simulink model "OML58_Cores2"  (R2021b)
settings: Solver=ode1  StartTime=0.0  StopTime=10  FixedStep=Ts  RelTol=1e-3
PostLoadFcn:
  | Ts = 50e-6;
InitFcn:
  | Ts = 50e-6;
undefined symbols (not defined in the file): I, Left, Right, type, V, X
libraries: spsSeriesRLCBranchLib x30, artemis x20, spsThreePhaseSeriesRLCBranchLib x19, spsThreePhaseSeriesRLCLoadLib x15, spsThreePhaseBreakerLib x15, spsGroundLib x12, rtlab x9, LafaeLib x8, spsThreePhaseVIMeasurementLib x7, spsThreePhaseTransformerTwoWindingsLib x5, spsPower3phInstantaneousLib x5, spsStairGeneratorLib x2
(part 3 of 3)

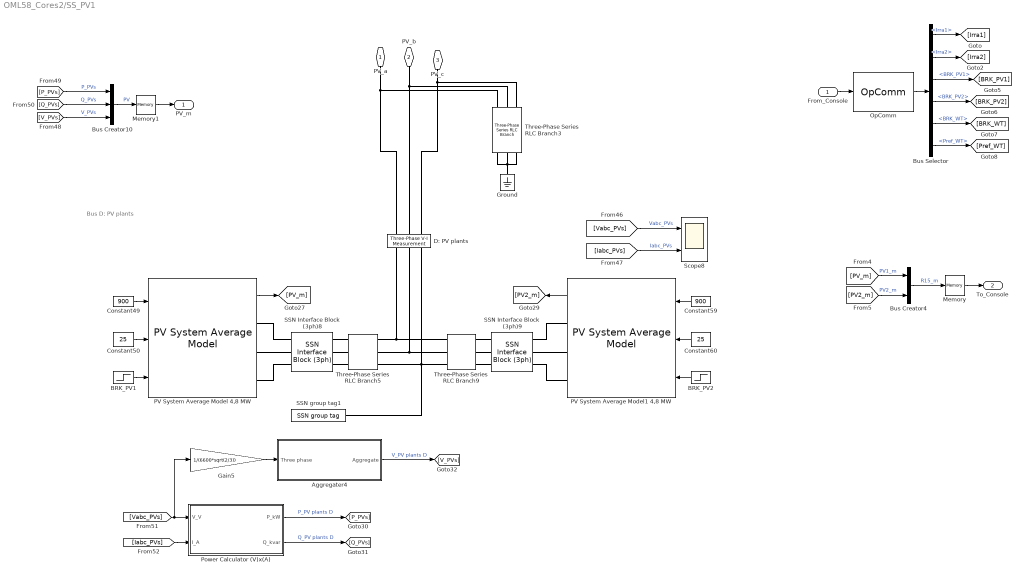
== system OML58_Cores2/SS_PV1 ==
  note: Bus D: PV plants
  From_Console : Inport
  Aggregater4 : Subsystem
      mask Display: image('$imagefile'); % Use "Edit Image" on toolstrip to change.
  BRK_PV1 : Step  Time=40  SampleTime=0
  BRK_PV2 : Step  Time=45  SampleTime=0
  Bus Creator10 : BusCreator  Inputs=3
  Bus Creator4 : BusCreator  Inputs=2
  Bus Selector : BusSelector  OutputSignals=Irra1,Irra2,BRK_PV1,BRK_PV2,BRK_WT,Pref_WT
  Constant49 : Constant  Value=900
  Constant50 : Constant  Value=25
  Constant59 : Constant  Value=900
  Constant60 : Constant  Value=25
  D: PV plants : spsThreePhaseVIMeasurementLib/Three-Phase V-I Measurement  VoltageMeasurement=phase-to-ground  SetLabelV=on  LabelV=Vabc_PVs  Vpu=off  VpuLL=off  CurrentMeasurement=yes  SetLabelI=on  LabelI=Iabc_PVs  Ipu=off  Pbase=100e6  Vbase=500e3  OutputType=Magnitude  PhasorSimulation=off  PSBequivalent=0
  Gain5 : Gain  Gain=1/(6600*sqrt(2/3))
  Ground : spsGroundLib/Ground  LConnTagsString=a
  Memory : Memory
  Memory1 : Memory
  OpComm : rtlab/OpComm  nbport=1  groupe_acq=1  subsys_rate=0  st=0  Synchronization=on  Interpolation=on  Threshold=1.0  Missed_Data=off  Sim_Time=off  Samples=off  dynSigOut=off  from_console=1  warning_done=off  writeOpCommFile=off  Offset=off
      settings: SourceProductName=RT-LAB
  PV System Average Model 4,8 MW : LafaeLib/PV System/PV System Average Model  Pnom=4.8e6  PF=1  fnom=50  Vdc_ref=1500  fsw=3*42*50  ripple_c=0.05  R1=0.001  Vdc_mpp=820.5  ripple_i_Boost=0.05  ripple_v_Boost=0.05  Vca_trafo_high=6.6e3  Vrms_high=6.6e3  Vrms_low=690  X_pu_trafo=0.1  tau_i=1e-3  Ts=Ts  Ts_Control=2*Ts
      link override PV Array: Npar=Np
      settings: SourceProductName=LAFAE Library
  PV System Average Model1 4,8 MW : LafaeLib/PV System/PV System Average Model  Pnom=4.8e6  PF=1  fnom=50  Vdc_ref=1500  fsw=3*42*50  ripple_c=0.05  R1=0.001  Vdc_mpp=820.5  ripple_i_Boost=0.05  ripple_v_Boost=0.05  Vca_trafo_high=6.6e3  Vrms_high=6.6e3  Vrms_low=690  X_pu_trafo=0.1  tau_i=1e-3  Ts=Ts  Ts_Control=2*Ts
      link override PV Array: Npar=Np
      settings: SourceProductName=LAFAE Library
  Power Calculator (V)x(A) : Subsystem
      mask DialogControl DescTextVar Prompt: Compute the three-phase instantaneous active and reactive powers associated with a periodic set of three-phase voltages and currents.
      mask DialogControl Control2 Prompt: Instantaneous reactive power is accurate only for balanced and harmonic-free three-phase voltages and currents.
      mask DialogControl Control3 Prompt: Current flowing into an RL circuit will produce positive active and reactive power.
      mask DialogControl Control4 Prompt: Input currents and voltages in (A) and (V), respectively.
      mask DialogControl Control5 Prompt: Output P and Q in kW and kvar, respectively.
      mask Display: image('$imagefile'); % Use "Edit Image" on toolstrip to change.
  SSN Interface Block (3ph)8 : artemis/SSN/Nodal Interface Blocks/SSN Interface Block (3ph)  nb_phase=3  nb_port=2  p1_type=I-type(Left)  p2_type=V-type (Right)  p3_type=V-type(Left)  p4_type=V-type(Left)  p5_type=V-type(Left)  p6_type=V-type(Left)  p7_type=V-type(Left)  p8_type=V-type(Left)  p9_type=V-type(Left)  p10_type=V-type(Left)  p11_type=V-type(Left)  p12_type=V-type(Left)  p13_type=V-type(Left)  p14_type=V-type(Left)  p15_type=V-type(Left)  p16_type=V-type(Left)  I_port_shunt_resistance=1e6
  SSN Interface Block (3ph)9 : artemis/SSN/Nodal Interface Blocks/SSN Interface Block (3ph)  nb_phase=3  nb_port=2  p1_type=V-type(Left)  p2_type=V-type (Right)  p3_type=V-type(Left)  p4_type=V-type(Left)  p5_type=V-type(Left)  p6_type=V-type(Left)  p7_type=V-type(Left)  p8_type=V-type(Left)  p9_type=V-type(Left)  p10_type=V-type(Left)  p11_type=V-type(Left)  p12_type=V-type(Left)  p13_type=V-type(Left)  p14_type=V-type(Left)  p15_type=V-type(Left)  p16_type=V-type(Left)  I_port_shunt_resistance=1e6
  SSN group tag1 : artemis/SSN/SSN group tag  ssn_group_tag=PV_Plant
  Scope8 : Scope  NumInputPorts=2
  Three-Phase Series RLC Branch3 : spsThreePhaseSeriesRLCBranchLib/Three-Phase Series RLC Branch  LConnTagsString=A|B|C  RConnTagsString=A|B|C  BranchType=L  Resistance=1  Inductance=2*2.5943  Capacitance=1e-6  Measurements=None
  Three-Phase Series RLC Branch5 : spsThreePhaseSeriesRLCBranchLib/Three-Phase Series RLC Branch  LConnTagsString=A|B|C  RConnTagsString=A|B|C  BranchType=R  Resistance=1e-6  Inductance=1e-3  Capacitance=1e-6  Measurements=None
  Three-Phase Series RLC Branch9 : spsThreePhaseSeriesRLCBranchLib/Three-Phase Series RLC Branch  LConnTagsString=A|B|C  RConnTagsString=A|B|C  BranchType=R  Resistance=1e-6  Inductance=1e-3  Capacitance=1e-6  Measurements=None
  PV_a : PMIOPort  Side=Right
  PV_b : PMIOPort  Port=2  Side=Right
  PV_c : PMIOPort  Port=3  Side=Right
  PV_m : Outport
  To_Console : Outport  Port=2
  wires:
  Memory/1 -> To_Console/1
  From_Console/1 -> OpComm/1
  OpComm/1 -> Bus Selector/1
  Bus Selector/1 -> [Irra1]  "<Irra1>"
  Bus Selector/2 -> [Irra2]  "<Irra2>"
  Bus Selector/3 -> [BRK_PV1]  "<BRK_PV1>"
  Bus Selector/4 -> [BRK_PV2]  "<BRK_PV2>"
  Bus Selector/5 -> [BRK_WT]  "<BRK_WT>"
  Bus Creator4/1 -> Memory/1  "R15_m"
  [PV2_m] -> Bus Creator4/2  "PV2_m"
  [PV_m] -> Bus Creator4/1  "PV1_m"
  Bus Selector/6 -> [Pref_WT]  "<Pref_WT>"
  BRK_PV2/1 -> PV System Average Model1 4,8 MW/3
  [V_PVs] -> Bus Creator10/3  "V_PVs"
  Gain5/1 -> Aggregater4/1(Three phase)
  [Vabc_PVs] -> Power Calculator (V)x(A)/1(V_V), Gain5/1
  Constant49/1 -> PV System Average Model 4,8 MW/1
  [Iabc_PVs] -> Scope8/2  "Iabc_PVs"
  Constant50/1 -> PV System Average Model 4,8 MW/2
  [Iabc_PVs] -> Power Calculator (V)x(A)/2(I_A)
  [Vabc_PVs] -> Scope8/1  "Vabc_PVs"
  Aggregater4/1(Aggregate) -> [V_PVs]  "V_PV plants D"
  Constant59/1 -> PV System Average Model1 4,8 MW/1
  BRK_PV1/1 -> PV System Average Model 4,8 MW/3
  Power Calculator (V)x(A)/2(Q_kvar) -> [Q_PVs]  "Q_PV plants D"
  Memory1/1 -> PV_m/1
  PV System Average Model1 4,8 MW/1 -> [PV2_m]
  Constant60/1 -> PV System Average Model1 4,8 MW/2
  Power Calculator (V)x(A)/1(P_kW) -> [P_PVs]  "P_PV plants D"
  Bus Creator10/1 -> Memory1/1  "PV"
  [P_PVs] -> Bus Creator10/1  "P_PVs"
  PV System Average Model 4,8 MW/1 -> [PV_m]
  [Q_PVs] -> Bus Creator10/2  "Q_PVs"
  connections:
  D: PV plants/RConn1 -- PV_a/RConn1 -- Three-Phase Series RLC Branch3/LConn1
  SSN group tag1/LConn1 -- D: PV plants/LConn3 -- Three-Phase Series RLC Branch5/LConn3 -- Three-Phase Series RLC Branch9/LConn3
  D: PV plants/RConn2 -- PV_b/RConn1 -- Three-Phase Series RLC Branch3/LConn2
  Three-Phase Series RLC Branch3/RConn1 -- Ground/LConn1 -- Three-Phase Series RLC Branch3/RConn2 -- Three-Phase Series RLC Branch3/RConn3
  D: PV plants/RConn3 -- PV_c/RConn1 -- Three-Phase Series RLC Branch3/LConn3
  Three-Phase Series RLC Branch9/LConn2 -- D: PV plants/LConn2 -- Three-Phase Series RLC Branch5/LConn2
  Three-Phase Series RLC Branch9/LConn1 -- D: PV plants/LConn1 -- Three-Phase Series RLC Branch5/LConn1
  Three-Phase Series RLC Branch5/RConn2 -- SSN Interface Block (3ph)8/LConn2
  PV System Average Model 4,8 MW/RConn3 -- SSN Interface Block (3ph)8/RConn3
  PV System Average Model 4,8 MW/RConn2 -- SSN Interface Block (3ph)8/RConn2
  PV System Average Model1 4,8 MW/RConn1 -- SSN Interface Block (3ph)9/LConn1
  SSN Interface Block (3ph)9/RConn1 -- Three-Phase Series RLC Branch9/RConn1
  Three-Phase Series RLC Branch5/RConn1 -- SSN Interface Block (3ph)8/LConn1
  SSN Interface Block (3ph)9/RConn2 -- Three-Phase Series RLC Branch9/RConn2
  SSN Interface Block (3ph)9/RConn3 -- Three-Phase Series RLC Branch9/RConn3
  PV System Average Model 4,8 MW/RConn1 -- SSN Interface Block (3ph)8/RConn1
  PV System Average Model1 4,8 MW/RConn2 -- SSN Interface Block (3ph)9/LConn2
  Three-Phase Series RLC Branch5/RConn3 -- SSN Interface Block (3ph)8/LConn3
  PV System Average Model1 4,8 MW/RConn3 -- SSN Interface Block (3ph)9/LConn3

== system OML58_Cores2/SM_powergrid/Aggregater ==
  Three phase : Inport
  Gain6 : Gain  Gain=2/3
  Sqrt : Sqrt  SaturateOnIntegerOverflow=on
  Square : Math  Operator=square  SaturateOnIntegerOverflow=on
  Sum5 : Sum  Inputs=1  CollapseMode=Specified dimension
  Aggregate : Outport
  wires:
  Gain6/1 -> Sqrt/1
  Sum5/1 -> Gain6/1
  Square/1 -> Sum5/1
  Sqrt/1 -> Aggregate/1
  Three phase/1 -> Square/1

== system OML58_Cores2/SM_powergrid/Aggregater1 ==
  Three phase : Inport
  Gain6 : Gain  Gain=2/3
  Sqrt : Sqrt  SaturateOnIntegerOverflow=on
  Square : Math  Operator=square  SaturateOnIntegerOverflow=on
  Sum5 : Sum  Inputs=1  CollapseMode=Specified dimension
  Aggregate : Outport
  wires:
  Gain6/1 -> Sqrt/1
  Sum5/1 -> Gain6/1
  Square/1 -> Sum5/1
  Sqrt/1 -> Aggregate/1
  Three phase/1 -> Square/1

== system OML58_Cores2/SM_powergrid/Aggregater2 ==
  Three phase : Inport
  Gain6 : Gain  Gain=2/3
  Sqrt : Sqrt  SaturateOnIntegerOverflow=on
  Square : Math  Operator=square  SaturateOnIntegerOverflow=on
  Sum5 : Sum  Inputs=1  CollapseMode=Specified dimension
  Aggregate : Outport
  wires:
  Gain6/1 -> Sqrt/1
  Sum5/1 -> Gain6/1
  Square/1 -> Sum5/1
  Sqrt/1 -> Aggregate/1
  Three phase/1 -> Square/1

== system OML58_Cores2/SM_powergrid/Aggregater3 ==
  Three phase : Inport
  Gain6 : Gain  Gain=2/3
  Sqrt : Sqrt  SaturateOnIntegerOverflow=on
  Square : Math  Operator=square  SaturateOnIntegerOverflow=on
  Sum5 : Sum  Inputs=1  CollapseMode=Specified dimension
  Aggregate : Outport
  wires:
  Gain6/1 -> Sqrt/1
  Sum5/1 -> Gain6/1
  Square/1 -> Sum5/1
  Sqrt/1 -> Aggregate/1
  Three phase/1 -> Square/1

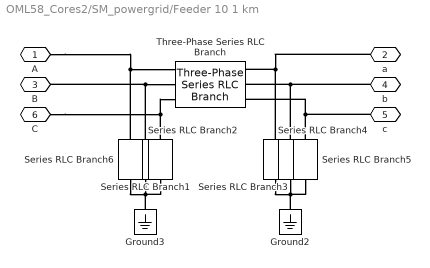
== system OML58_Cores2/SM_powergrid/Feeder 10 1 km ==
  Ground2 : spsGroundLib/Ground  LConnTagsString=a
  Ground3 : spsGroundLib/Ground  LConnTagsString=a
  Series RLC Branch{1..6} (6 alike) : spsSeriesRLCBranchLib/Series RLC Branch  LConnTagsString=__new0  RConnTagsString=__new0  BranchType=C  Resistance=1  Inductance=1e-3  SetiL0=off  InitialCurrent=0  Capacitance=l*0.495e-6/2  Setx0=off  InitialVoltage=0  Measurements=None
  Three-Phase Series RLC Branch : spsThreePhaseSeriesRLCBranchLib/Three-Phase Series RLC Branch  LConnTagsString=A|B|C  RConnTagsString=A|B|C  BranchType=RL  Resistance=l*0.0991  Inductance=l*0.602e-3  Capacitance=1e-6  Measurements=None
  A : PMIOPort  Side=Left
  a : PMIOPort  Port=2  Side=Right
  B : PMIOPort  Port=3  Side=Left
  b : PMIOPort  Port=4  Side=Right
  c : PMIOPort  Port=5  Side=Right
  C : PMIOPort  Port=6  Side=Left
  connections:
  Ground2/LConn1 -- Series RLC Branch5/RConn1 -- Series RLC Branch4/RConn1 -- Series RLC Branch3/RConn1
  Series RLC Branch2/LConn1 -- C/RConn1 -- Three-Phase Series RLC Branch/LConn3
  Ground3/LConn1 -- Series RLC Branch2/RConn1 -- Series RLC Branch1/RConn1 -- Series RLC Branch6/RConn1
  Series RLC Branch3/LConn1 -- a/RConn1 -- Three-Phase Series RLC Branch/RConn1
  Series RLC Branch6/LConn1 -- A/RConn1 -- Three-Phase Series RLC Branch/LConn1
  Series RLC Branch4/LConn1 -- b/RConn1 -- Three-Phase Series RLC Branch/RConn2
  Series RLC Branch5/LConn1 -- c/RConn1 -- Three-Phase Series RLC Branch/RConn3
  Series RLC Branch1/LConn1 -- B/RConn1 -- Three-Phase Series RLC Branch/LConn2

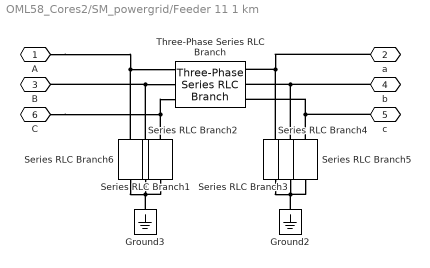
== system OML58_Cores2/SM_powergrid/Feeder 11 1 km ==
  Ground2 : spsGroundLib/Ground  LConnTagsString=a
  Ground3 : spsGroundLib/Ground  LConnTagsString=a
  Series RLC Branch{1..6} (6 alike) : spsSeriesRLCBranchLib/Series RLC Branch  LConnTagsString=__new0  RConnTagsString=__new0  BranchType=C  Resistance=1  Inductance=1e-3  SetiL0=off  InitialCurrent=0  Capacitance=l*0.495e-6/2  Setx0=off  InitialVoltage=0  Measurements=None
  Three-Phase Series RLC Branch : spsThreePhaseSeriesRLCBranchLib/Three-Phase Series RLC Branch  LConnTagsString=A|B|C  RConnTagsString=A|B|C  BranchType=RL  Resistance=l*0.0991  Inductance=l*0.602e-3  Capacitance=1e-6  Measurements=None
  A : PMIOPort  Side=Left
  a : PMIOPort  Port=2  Side=Right
  B : PMIOPort  Port=3  Side=Left
  b : PMIOPort  Port=4  Side=Right
  c : PMIOPort  Port=5  Side=Right
  C : PMIOPort  Port=6  Side=Left
  connections:
  Ground2/LConn1 -- Series RLC Branch5/RConn1 -- Series RLC Branch4/RConn1 -- Series RLC Branch3/RConn1
  Series RLC Branch2/LConn1 -- C/RConn1 -- Three-Phase Series RLC Branch/LConn3
  Ground3/LConn1 -- Series RLC Branch2/RConn1 -- Series RLC Branch1/RConn1 -- Series RLC Branch6/RConn1
  Series RLC Branch3/LConn1 -- a/RConn1 -- Three-Phase Series RLC Branch/RConn1
  Series RLC Branch6/LConn1 -- A/RConn1 -- Three-Phase Series RLC Branch/LConn1
  Series RLC Branch4/LConn1 -- b/RConn1 -- Three-Phase Series RLC Branch/RConn2
  Series RLC Branch5/LConn1 -- c/RConn1 -- Three-Phase Series RLC Branch/RConn3
  Series RLC Branch1/LConn1 -- B/RConn1 -- Three-Phase Series RLC Branch/LConn2

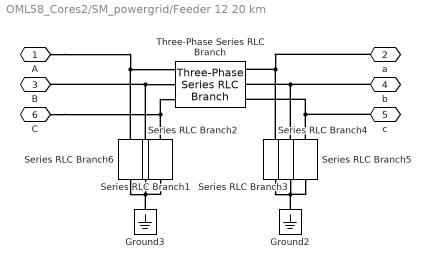
== system OML58_Cores2/SM_powergrid/Feeder 12 20 km ==
  Ground2 : spsGroundLib/Ground  LConnTagsString=a
  Ground3 : spsGroundLib/Ground  LConnTagsString=a
  Series RLC Branch{1..6} (6 alike) : spsSeriesRLCBranchLib/Series RLC Branch  LConnTagsString=__new0  RConnTagsString=__new0  BranchType=C  Resistance=1  Inductance=1e-3  SetiL0=off  InitialCurrent=0  Capacitance=l*0.495e-6/2  Setx0=off  InitialVoltage=0  Measurements=None
  Three-Phase Series RLC Branch : spsThreePhaseSeriesRLCBranchLib/Three-Phase Series RLC Branch  LConnTagsString=A|B|C  RConnTagsString=A|B|C  BranchType=RL  Resistance=l*0.0991  Inductance=l*0.602e-3  Capacitance=1e-6  Measurements=None
  A : PMIOPort  Side=Left
  a : PMIOPort  Port=2  Side=Right
  B : PMIOPort  Port=3  Side=Left
  b : PMIOPort  Port=4  Side=Right
  c : PMIOPort  Port=5  Side=Right
  C : PMIOPort  Port=6  Side=Left
  connections:
  Ground2/LConn1 -- Series RLC Branch5/RConn1 -- Series RLC Branch4/RConn1 -- Series RLC Branch3/RConn1
  Series RLC Branch2/LConn1 -- C/RConn1 -- Three-Phase Series RLC Branch/LConn3
  Ground3/LConn1 -- Series RLC Branch2/RConn1 -- Series RLC Branch1/RConn1 -- Series RLC Branch6/RConn1
  Series RLC Branch3/LConn1 -- a/RConn1 -- Three-Phase Series RLC Branch/RConn1
  Series RLC Branch6/LConn1 -- A/RConn1 -- Three-Phase Series RLC Branch/LConn1
  Series RLC Branch4/LConn1 -- b/RConn1 -- Three-Phase Series RLC Branch/RConn2
  Series RLC Branch5/LConn1 -- c/RConn1 -- Three-Phase Series RLC Branch/RConn3
  Series RLC Branch1/LConn1 -- B/RConn1 -- Three-Phase Series RLC Branch/LConn2

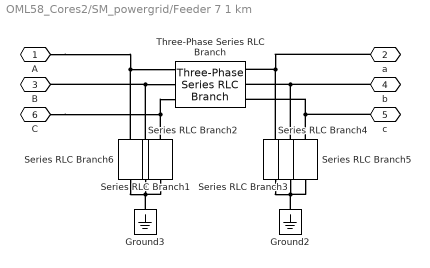
== system OML58_Cores2/SM_powergrid/Feeder 7 1 km ==
  Ground2 : spsGroundLib/Ground  LConnTagsString=a
  Ground3 : spsGroundLib/Ground  LConnTagsString=a
  Series RLC Branch{1..6} (6 alike) : spsSeriesRLCBranchLib/Series RLC Branch  LConnTagsString=__new0  RConnTagsString=__new0  BranchType=C  Resistance=1  Inductance=1e-3  SetiL0=off  InitialCurrent=0  Capacitance=l*0.495e-6/2  Setx0=off  InitialVoltage=0  Measurements=None
  Three-Phase Series RLC Branch : spsThreePhaseSeriesRLCBranchLib/Three-Phase Series RLC Branch  LConnTagsString=A|B|C  RConnTagsString=A|B|C  BranchType=RL  Resistance=l*0.0991  Inductance=l*0.602e-3  Capacitance=1e-6  Measurements=None
  A : PMIOPort  Side=Left
  a : PMIOPort  Port=2  Side=Right
  B : PMIOPort  Port=3  Side=Left
  b : PMIOPort  Port=4  Side=Right
  c : PMIOPort  Port=5  Side=Right
  C : PMIOPort  Port=6  Side=Left
  connections:
  Ground2/LConn1 -- Series RLC Branch5/RConn1 -- Series RLC Branch4/RConn1 -- Series RLC Branch3/RConn1
  Series RLC Branch2/LConn1 -- C/RConn1 -- Three-Phase Series RLC Branch/LConn3
  Ground3/LConn1 -- Series RLC Branch2/RConn1 -- Series RLC Branch1/RConn1 -- Series RLC Branch6/RConn1
  Series RLC Branch3/LConn1 -- a/RConn1 -- Three-Phase Series RLC Branch/RConn1
  Series RLC Branch6/LConn1 -- A/RConn1 -- Three-Phase Series RLC Branch/LConn1
  Series RLC Branch4/LConn1 -- b/RConn1 -- Three-Phase Series RLC Branch/RConn2
  Series RLC Branch5/LConn1 -- c/RConn1 -- Three-Phase Series RLC Branch/RConn3
  Series RLC Branch1/LConn1 -- B/RConn1 -- Three-Phase Series RLC Branch/LConn2

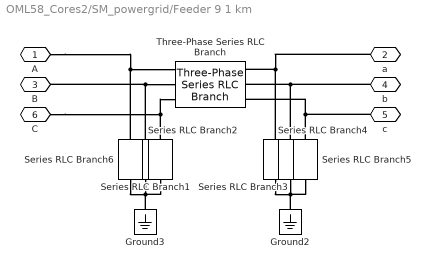
== system OML58_Cores2/SM_powergrid/Feeder 9 1 km ==
  Ground2 : spsGroundLib/Ground  LConnTagsString=a
  Ground3 : spsGroundLib/Ground  LConnTagsString=a
  Series RLC Branch{1..6} (6 alike) : spsSeriesRLCBranchLib/Series RLC Branch  LConnTagsString=__new0  RConnTagsString=__new0  BranchType=C  Resistance=1  Inductance=1e-3  SetiL0=off  InitialCurrent=0  Capacitance=l*0.495e-6/2  Setx0=off  InitialVoltage=0  Measurements=None
  Three-Phase Series RLC Branch : spsThreePhaseSeriesRLCBranchLib/Three-Phase Series RLC Branch  LConnTagsString=A|B|C  RConnTagsString=A|B|C  BranchType=RL  Resistance=l*0.0991  Inductance=l*0.602e-3  Capacitance=1e-6  Measurements=None
  A : PMIOPort  Side=Left
  a : PMIOPort  Port=2  Side=Right
  B : PMIOPort  Port=3  Side=Left
  b : PMIOPort  Port=4  Side=Right
  c : PMIOPort  Port=5  Side=Right
  C : PMIOPort  Port=6  Side=Left
  connections:
  Ground2/LConn1 -- Series RLC Branch5/RConn1 -- Series RLC Branch4/RConn1 -- Series RLC Branch3/RConn1
  Series RLC Branch2/LConn1 -- C/RConn1 -- Three-Phase Series RLC Branch/LConn3
  Ground3/LConn1 -- Series RLC Branch2/RConn1 -- Series RLC Branch1/RConn1 -- Series RLC Branch6/RConn1
  Series RLC Branch3/LConn1 -- a/RConn1 -- Three-Phase Series RLC Branch/RConn1
  Series RLC Branch6/LConn1 -- A/RConn1 -- Three-Phase Series RLC Branch/LConn1
  Series RLC Branch4/LConn1 -- b/RConn1 -- Three-Phase Series RLC Branch/RConn2
  Series RLC Branch5/LConn1 -- c/RConn1 -- Three-Phase Series RLC Branch/RConn3
  Series RLC Branch1/LConn1 -- B/RConn1 -- Three-Phase Series RLC Branch/LConn2

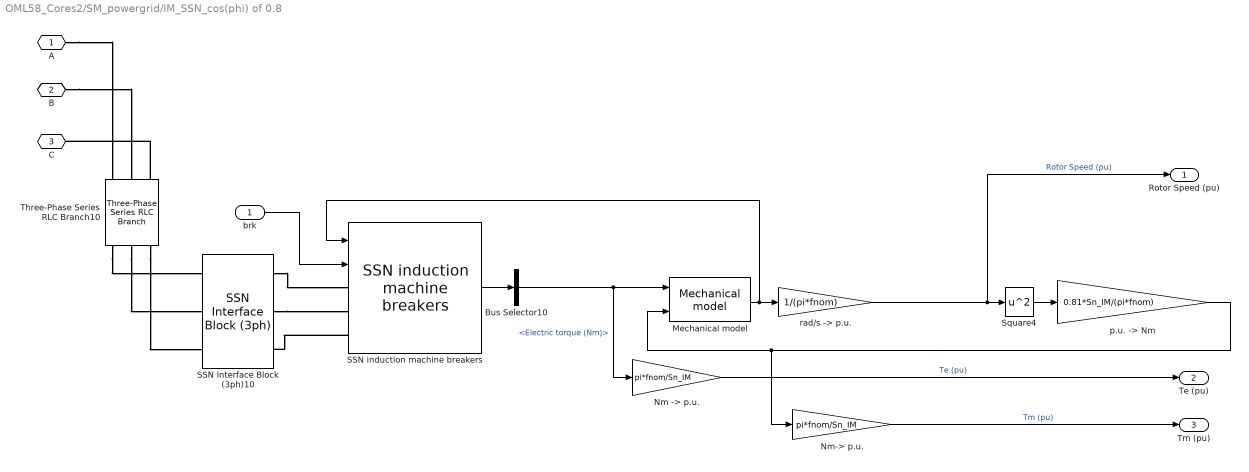
== system OML58_Cores2/SM_powergrid/IM_SSN_cos(phi) of 0.8 ==
  brk : Inport
  Bus Selector10 : BusSelector  OutputSignals=Electric torque (Nm)
  Mechanical model : artemis/SSN/SSN rotating machines/Mechanical model  J=Sn_IM/(fnom*pi)^2  F=6.2988e-004  fo=eps  Ts=Ts
  "Nm -> p.u." : Gain  Gain=pi*fnom/Sn_IM
  Nm-> p.u. : Gain  Gain=pi*fnom/Sn_IM
  SSN Interface Block (3ph)10 : artemis/SSN/Nodal Interface Blocks/SSN Interface Block (3ph)  nb_phase=3  nb_port=2  p1_type=X-type(Right)  p2_type=V-type(Left)  p3_type=V-type(Left)  p4_type=V-type(Left)  p5_type=V-type(Left)  p6_type=V-type(Left)  p7_type=V-type(Left)  p8_type=V-type(Left)  p9_type=V-type(Left)  p10_type=V-type(Left)  p11_type=V-type(Left)  p12_type=V-type(Left)  p13_type=V-type(Left)  p14_type=V-type(Left)  p15_type=V-type(Left)  p16_type=V-type(Left)  I_port_shunt_resistance=1e9
  SSN induction machine breakers : artemis/SSN/SSN rotating machines/SSN induction machine breakers  Rs=0.01965*Vac^2/Sn_IM  Lls=0.0397*Vac^2/(Sn_IM*fnom*2*pi)  Rr=0.01909*Vac^2/Sn_IM  Llr=0.0397*Vac^2/(Sn_IM*fnom*2*pi)  Lm=1.75*Vac^2/(Sn_IM*fnom*2*pi)  pp=2  Ts=Ts  nnode=3  taggg=72fx9e34x6e280f1ea945  be_option=off  Roff=1e6  Ron=1e-3
  Square4 : Math  Operator=square  SaturateOnIntegerOverflow=on
  Three-Phase Series RLC Branch10 : spsThreePhaseSeriesRLCBranchLib/Three-Phase Series RLC Branch  LConnTagsString=A|B|C  RConnTagsString=A|B|C  BranchType=R  Resistance=1e-6  Inductance=1e-3  Capacitance=1e-6  Measurements=None
  "p.u. -> Nm" : Gain  Gain=0.81*Sn_IM/(pi*fnom)
  "rad/s -> p.u." : Gain  Gain=1/(pi*fnom)
  A : PMIOPort  Side=Left
  B : PMIOPort  Port=2  Side=Left
  C : PMIOPort  Port=3  Side=Left
  Rotor Speed (pu) : Outport
  Te (pu) : Outport  Port=2
  Tm (pu) : Outport  Port=3
  wires:
  "rad/s -> p.u."/1 -> Rotor Speed (pu)/1, Square4/1  "Rotor Speed (pu)"
  Mechanical model/1 -> SSN induction machine breakers/1, "rad/s -> p.u."/1
  brk/1 -> SSN induction machine breakers/2
  SSN induction machine breakers/1 -> Bus Selector10/1
  "p.u. -> Nm"/1 -> Mechanical model/2, Nm-> p.u./1
  Bus Selector10/1 -> "Nm -> p.u."/1, Mechanical model/1  "<Electric torque (Nm)>"
  Square4/1 -> "p.u. -> Nm"/1
  Nm-> p.u./1 -> Tm (pu)/1  "Tm (pu)"
  "Nm -> p.u."/1 -> Te (pu)/1  "Te (pu)"
  connections:
  Three-Phase Series RLC Branch10/RConn3 -- SSN Interface Block (3ph)10/LConn3
  SSN induction machine breakers/LConn3 -- SSN Interface Block (3ph)10/RConn3
  B/RConn1 -- Three-Phase Series RLC Branch10/LConn2
  Three-Phase Series RLC Branch10/RConn2 -- SSN Interface Block (3ph)10/LConn2
  SSN Interface Block (3ph)10/RConn1 -- SSN induction machine breakers/LConn1
  SSN Interface Block (3ph)10/RConn2 -- SSN induction machine breakers/LConn2
  Three-Phase Series RLC Branch10/RConn1 -- SSN Interface Block (3ph)10/LConn1
  A/RConn1 -- Three-Phase Series RLC Branch10/LConn1
  Three-Phase Series RLC Branch10/LConn3 -- C/RConn1

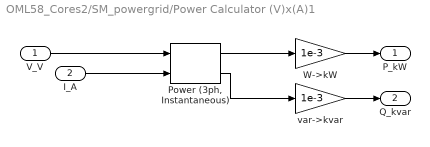
== system OML58_Cores2/SM_powergrid/Power Calculator (V)x(A)1 ==
  V_V : Inport
  I_A : Inport  Port=2
  "Power (3ph, Instantaneous)" : spsPower3phInstantaneousLib/Power (3ph, Instantaneous)
  W->kW : Gain  Gain=1e-3
  var->kvar : Gain  Gain=1e-3
  P_kW : Outport
  Q_kvar : Outport  Port=2
  wires:
  V_V/1 -> "Power (3ph, Instantaneous)"/1
  I_A/1 -> "Power (3ph, Instantaneous)"/2
  "Power (3ph, Instantaneous)"/1 -> W->kW/1
  "Power (3ph, Instantaneous)"/2 -> var->kvar/1
  W->kW/1 -> P_kW/1
  var->kvar/1 -> Q_kvar/1

== system OML58_Cores2/SM_powergrid/Power Calculator (V)x(A)2 ==
  V_V : Inport
  I_A : Inport  Port=2
  "Power (3ph, Instantaneous)" : spsPower3phInstantaneousLib/Power (3ph, Instantaneous)
  W->kW : Gain  Gain=1e-3
  var->kvar : Gain  Gain=1e-3
  P_kW : Outport
  Q_kvar : Outport  Port=2
  wires:
  V_V/1 -> "Power (3ph, Instantaneous)"/1
  I_A/1 -> "Power (3ph, Instantaneous)"/2
  "Power (3ph, Instantaneous)"/1 -> W->kW/1
  "Power (3ph, Instantaneous)"/2 -> var->kvar/1
  W->kW/1 -> P_kW/1
  var->kvar/1 -> Q_kvar/1

== system OML58_Cores2/SM_powergrid/Power Calculator (V)x(A)3 ==
  V_V : Inport
  I_A : Inport  Port=2
  "Power (3ph, Instantaneous)" : spsPower3phInstantaneousLib/Power (3ph, Instantaneous)
  W->kW : Gain  Gain=1e-3
  var->kvar : Gain  Gain=1e-3
  P_kW : Outport
  Q_kvar : Outport  Port=2
  wires:
  V_V/1 -> "Power (3ph, Instantaneous)"/1
  I_A/1 -> "Power (3ph, Instantaneous)"/2
  "Power (3ph, Instantaneous)"/1 -> W->kW/1
  "Power (3ph, Instantaneous)"/2 -> var->kvar/1
  W->kW/1 -> P_kW/1
  var->kvar/1 -> Q_kvar/1

== system OML58_Cores2/SM_powergrid/Power Calculator (V)x(A)4 ==
  V_V : Inport
  I_A : Inport  Port=2
  "Power (3ph, Instantaneous)" : spsPower3phInstantaneousLib/Power (3ph, Instantaneous)
  W->kW : Gain  Gain=1e-3
  var->kvar : Gain  Gain=1e-3
  P_kW : Outport
  Q_kvar : Outport  Port=2
  wires:
  V_V/1 -> "Power (3ph, Instantaneous)"/1
  I_A/1 -> "Power (3ph, Instantaneous)"/2
  "Power (3ph, Instantaneous)"/1 -> W->kW/1
  "Power (3ph, Instantaneous)"/2 -> var->kvar/1
  W->kW/1 -> P_kW/1
  var->kvar/1 -> Q_kvar/1

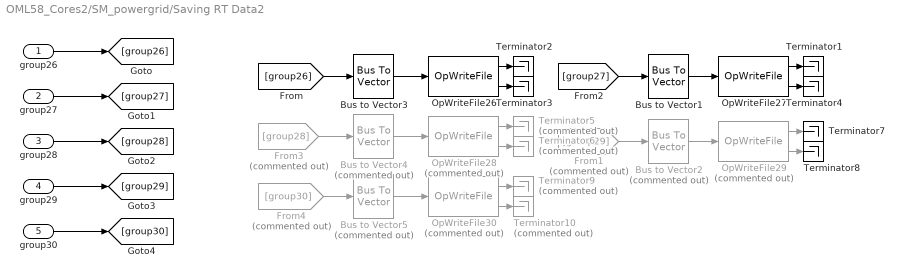
== system OML58_Cores2/SM_powergrid/Saving RT Data2 ==
  group26 : Inport
  group27 : Inport  Port=2
  group28 : Inport  Port=3
  group29 : Inport  Port=4
  group30 : Inport  Port=5
  Bus to Vector1 : BusToVector
  Bus to Vector2 : BusToVector  Commented=on
  Bus to Vector3 : BusToVector
  Bus to Vector4 : BusToVector  Commented=on
  Bus to Vector5 : BusToVector  Commented=on
  From1 : From  Commented=on  GotoTag=group29
  From3 : From  Commented=on  GotoTag=group28
  From4 : From  Commented=on  GotoTag=group30
  OpWriteFile26 : rtlab/DataLogging/OpWriteFile  Static_File=on  varname=Sources_m  Filename=Sources_m.mat  rtpath='./'  nrtpath='.\'  Acq_Group=26  file_size=(nls26+1)*8*(ld26/Ts)*1.5  write_offline=on  Sim_Mode=off  Nb_Samples=ld26/Ts  Buffer_size=(ld26/Ts)*8*(1+nls26)
      settings: SourceProductName=RT-LAB  Decimation=Decimation26
  OpWriteFile27 : rtlab/DataLogging/OpWriteFile  Static_File=on  varname=Loads_m  Filename=Loads_m.mat  rtpath='./'  nrtpath='.\'  Acq_Group=27  file_size=(nls27+1)*8*(ld27/Ts)*1.5  write_offline=on  Sim_Mode=off  Nb_Samples=ld27/Ts  Buffer_size=(ld26/Ts)*8*(1+nls26)
      settings: SourceProductName=RT-LAB  Decimation=Decimation27
  OpWriteFile28 : rtlab/DataLogging/OpWriteFile  Commented=on  Static_File=on  varname=Meas_Q  Filename=Meas_Q.mat  rtpath='./'  nrtpath='.\'  Acq_Group=28  file_size=(nls28+1)*8*(ld28/Ts)*1.5  write_offline=on  Sim_Mode=off  Nb_Samples=ld28/Ts  Buffer_size=(ld28/Ts)*8*(1+nls28)
      settings: SourceProductName=RT-LAB  Decimation=Decimation28
  OpWriteFile29 : rtlab/DataLogging/OpWriteFile  Commented=on  Static_File=on  varname=P_Loads  Filename=P_Loads.mat  rtpath='./'  nrtpath='.\'  Acq_Group=29  file_size=(nls29+1)*8*(ld29/Ts)*1.5  write_offline=on  Sim_Mode=off  Nb_Samples=ld29/Ts  Buffer_size=(ld29/Ts)*8*(1+nls29)
      settings: SourceProductName=RT-LAB  Decimation=Decimation29
  OpWriteFile30 : rtlab/DataLogging/OpWriteFile  Commented=on  Static_File=on  varname=Q_Loads  Filename=Q_Loads.mat  rtpath='./'  nrtpath='.\'  Acq_Group=30  file_size=(nls30+1)*8*(ld30/Ts)*1.5  write_offline=on  Sim_Mode=off  Nb_Samples=ld30/Ts  Buffer_size=(ld30/Ts)*8*(1+nls30)
      settings: SourceProductName=RT-LAB  Decimation=Decimation30
  Terminator{1..4,7..8} (6 alike) : Terminator
  Terminator{5..6,9..10} (4 alike) : Terminator  Commented=on
  wires:
  OpWriteFile28/2 -> Terminator6/1
  OpWriteFile27/1 -> Terminator1/1
  OpWriteFile26/2 -> Terminator3/1
  OpWriteFile26/1 -> Terminator2/1
  OpWriteFile30/1 -> Terminator9/1
  OpWriteFile27/2 -> Terminator4/1
  OpWriteFile29/2 -> Terminator8/1
  OpWriteFile30/2 -> Terminator10/1
  OpWriteFile29/1 -> Terminator7/1
  OpWriteFile28/1 -> Terminator5/1
  group26/1 -> [group26]
  group27/1 -> [group27]
  group28/1 -> [group28]
  group29/1 -> [group29]
  group30/1 -> [group30]
  [group27] -> Bus to Vector1/1
  Bus to Vector1/1 -> OpWriteFile27/1
  From1/1 -> Bus to Vector2/1
  Bus to Vector2/1 -> OpWriteFile29/1
  [group26] -> Bus to Vector3/1
  Bus to Vector3/1 -> OpWriteFile26/1
  From3/1 -> Bus to Vector4/1
  Bus to Vector4/1 -> OpWriteFile28/1
  From4/1 -> Bus to Vector5/1
  Bus to Vector5/1 -> OpWriteFile30/1

== system OML58_Cores2/SS_PV1/Aggregater4 ==
  Three phase : Inport
  Gain6 : Gain  Gain=2/3
  Sqrt : Sqrt  SaturateOnIntegerOverflow=on
  Square : Math  Operator=square  SaturateOnIntegerOverflow=on
  Sum5 : Sum  Inputs=1  CollapseMode=Specified dimension
  Aggregate : Outport
  wires:
  Gain6/1 -> Sqrt/1
  Sum5/1 -> Gain6/1
  Square/1 -> Sum5/1
  Sqrt/1 -> Aggregate/1
  Three phase/1 -> Square/1

== system OML58_Cores2/SS_PV1/Power Calculator (V)x(A) ==
  V_V : Inport
  I_A : Inport  Port=2
  "Power (3ph, Instantaneous)" : spsPower3phInstantaneousLib/Power (3ph, Instantaneous)
  W->kW : Gain  Gain=1e-3
  var->kvar : Gain  Gain=1e-3
  P_kW : Outport
  Q_kvar : Outport  Port=2
  wires:
  V_V/1 -> "Power (3ph, Instantaneous)"/1
  I_A/1 -> "Power (3ph, Instantaneous)"/2
  "Power (3ph, Instantaneous)"/1 -> W->kW/1
  "Power (3ph, Instantaneous)"/2 -> var->kvar/1
  W->kW/1 -> P_kW/1
  var->kvar/1 -> Q_kvar/1
